simulink model "e8_IPMSM_HWJandVent_ROM"  (R2021b)
settings: Solver=VariableStepAuto  StartTime=0.0  StopTime=1000  RelTol=1e-3  AbsTol=1e-3
model workspace (MAT data in the model file):
  AdjacencyMat = [0 0 0 0 0 0 0 0 0 0 0 0 ... (15129 elements, 123x123)]
  Banding_Loss_Mat = [0 0 0 0 0 0 0 0 0 0 0 0 ... (7020 elements, 39x60x3)]
  CapMat = [1e+20; 2196.70091586; 387.653102799; 193.8265514; 1962.34710525; 387.653102799; 193.8265514; 1962.34710525; 1266.59353814; 268.053957132; 416.539515956; 175.715078; 577.243160678; 310.101557898; 23.9530731873; 15.4990473565; 47.9061463746; 30.998094713; 85.98384; 1.11955442905; 1.11955442905; 1.11955442905; 1.11955442905; 1.11955442905; 1.11955442905; 0.373184809682; 0.373184809682; 450.202206395; 54.9511679003; 54.9511679003; 247.389926005; 247.389926005; 75.306462; 75.306462; 1.11955442905; 1.11955442905; 1e+20; 1e+20; 0; 0; 0; 0; 429.469897824; 0; 0; 0; 0; 429.469897824; 0; 0; 0; 0; 0; 0; 424.408023296; 268.053957132; 0; 0; 0; 0; 0; 322.102423368; 0; 0; 0; 0; 0; 322.102423368; 0; 0; 0; 0; 0; 318.306017472; 268.053957132; 2196.70091586; 1266.59353814; 268.053957132; 416.539515956; 175.715078; 577.243160678; 310.101557898; 85.98384; 0.373184809682; 0.373184809682; 450.202206395; 0; 0; 0; 0; 0; 424.408023296; 268.053957132; 0; 0; 0; 0; 318.306017472; 268.053957132; 2196.70091586; 1266.59353814; 268.053957132; 416.539515956; 175.715078; 577.243160678; 310.101557898; 85.98384; 0.373184809682; 0.373184809682; 450.202206395; 0; 0; 0; 0; 0; 424.408023296; 268.053957132; 0; 0; 0; 0; 318.306017472; 268.053957132]
  CoolantArrayIdxs = [20; 21; 22; 23; 24; 25; 26; 27; 35; 36; 37; 84; 85; 108; 109; 19; 38; 83; 107]
  DCBusVoltageVec = [200 300 400]
  Friction_Loss_Mat = [0 0 0 0 0 0 0 0 0 0 0 0 ... (7020 elements, 39x60x3)]
  InletCoolIdxs = [38; 37]
  Iron_Loss_Rotor_Back_Iron_Mat = [0.0117705351991 0.0204390240307 0.0248508325185 0.0256457032681 0.0238785055856 0.020530699908 0.0166089076031 0.0132296142351 0.0115805086727 0.0121981902442 0.0144548234671 0.0172622621719 ... (7020 elements, 39x60x3)]
  Iron_Loss_Rotor_Pole_Mat = [1.45649756865 1.45220158629 1.42754923451 1.38825604934 1.33915333349 1.28386605183 1.22530180492 1.16593914393 1.10785564554 1.05188090135 0.997097257278 0.941639677474 ... (7020 elements, 39x60x3)]
  Iron_Loss_Rotor_Tooth_Mat = [0 0 0 0 0 0 0 0 0 0 0 0 ... (7020 elements, 39x60x3)]
  Iron_Loss_Stator_Back_Iron_Mat = [38.5419456951 37.7152025365 36.7151009719 35.6149517682 34.4520386289 33.2585547415 32.0665067995 30.91142079 29.8301048499 28.8255844376 27.8319778373 26.7434652419 ... (7020 elements, 39x60x3)]
  Iron_Loss_Stator_Tooth_Mat = [42.0610884508 40.9832240847 40.1258499541 39.3817529075 38.6582544091 37.9130136221 37.1370624807 36.3449214788 35.5617649366 34.7840580455 33.951564889 32.9872940506 ... (7020 elements, 39x60x3)]
  LossDistrForEachType = [0 0 0 0 0 0 0 0 0 0 0 0 ... (2952 elements, 24x123)]
  Magnet_Loss_Mat = [0.0995193918038 0.0923780277949 0.0864844160887 0.0815810725061 0.0772064600726 0.0729767275694 0.0685055432332 0.0633314716331 0.0569179480863 0.0491401889658 0.0406359949749 0.0323130751847 ... (7020 elements, 39x60x3)]
  OutletCoolIdxs = [107  107  107; 20  22  23]
  RotorCopperTempCoefResistivity = 0.00393
  Rotor_Cage_Loss_Mat = [0 0 0 0 0 0 0 0 0 0 0 0 ... (7020 elements, 39x60x3)]
  ShaftTorqueVec = [-286.936099977 -271.951133863 -256.966167748 -241.981201634 -226.99623552 -212.011269406 -197.026303292 -182.041337178 -167.056371063 -152.071404949 -137.086438835 -122.101472721 -107.116506607 -92.1315404924 -77.1465743783 -62.1616082641 -47.1766421499 -32.1916760357 -17.2067099215 -2.22174380736 12.7632223068 27.748188421 42.7331545352 57.7181206494 72.7030867635 87.6880528777 102.673018992 117.657985106 132.64295122 147.627917334 162.612883449 177.597849563 192.582815677 207.567781791 222.552747905 237.53771402 252.522680134 267.507646248 282.492612362]
  Sleeve_Loss_Mat = [0 0 0 0 0 0 0 0 0 0 0 0 ... (7020 elements, 39x60x3)]
  SpeedVec = [500 661.016949153 822.033898305 983.050847458 1144.06779661 1305.08474576 1466.10169492 1627.11864407 1788.13559322 1949.15254237 2110.16949153 2271.18644068 2432.20338983 2593.22033898 2754.23728814 2915.25423729 3076.27118644 3237.28813559 3398.30508475 3559.3220339 3720.33898305 3881.3559322 4042.37288136 4203.38983051 4364.40677966 4525.42372881 4686.44067797 4847.45762712 5008.47457627 5169.49152542 5330.50847458 5491.52542373 5652.54237288 5813.55932203 5974.57627119 6135.59322034 6296.61016949 6457.62711864 6618.6440678 6779.66101695 6940.6779661 7101.69491525 7262.71186441 7423.72881356 7584.74576271 7745.76271186 7906.77966102 8067.79661017 8228.81355932 8389.83050847 8550.84745763 8711.86440678 8872.88135593 9033.89830508 9194.91525424 9355.93220339 9516.94915254 9677.96610169 9838.98305085 10000]
  StateSpaceND : object (value not decoded)
  StatorCopperTempCoefResistivity = 0.00393
  Stator_Copper_Loss_AC_Mat = [0 0 0 0 0 0 0 0 0 0 0 0 ... (7020 elements, 39x60x3)]
  Stator_Copper_Loss_Mat = [3925.33912093 3478.13441392 3061.95534758 2688.26015542 2350.64396183 2044.39353286 1765.95289325 1512.57803512 1282.11615226 1072.87404999 883.521113045 712.988793321 ... (7020 elements, 39x60x3)]
  Stray_Load_Loss_Mat = [0 0 0 0 0 0 0 0 0 0 0 0 ... (7020 elements, 39x60x3)]
  Stray_Loss_Stator_Iron_Proportion = 0.95
  TnodesInit = [25; 25; 25; 25; 25; 25; 25; 25; 25; 25; 25; 25; 25; 25; 25; 25; 25; 25; 25; 25; 25; 25; 25; 25; 25; 25; 25; 25; 25; 25; 25; 25; 25; 25; 25; 25; 25; 25; 25; 25; 25; 25; 25; 25; 25; 25; 25; 25; 25; 25; 25; 25; 25; 25; 25; 25; 25; 25; 25; 25; 25; 25; 25; 25; 25; 25; 25; 25; 25; 25; 25; 25; 25; 25; 25; 25; 25; 25; 25; 25; 25; 25; 25; 25; 25; 25; 25; 25; 25; 25; 25; 25; 25; 25; 25; 25; 25; 25; 25; 25; 25; 25; 25; 25; 25; 25; 25; 25; 25; 25; 25; 25; 25; 25; 25; 25; 25; 25; 25; 25; 25; 25; 25]
  TrefRotor = 20
  TrefStator = 20
  Windage_Loss_Mat = [0 0 0 0 0 0 0 0 0 0 0 0 ... (7020 elements, 39x60x3)]
libraries: mcadROM_lib x4
(part 1 of 2)
settings Model: Creator=agonzale  LastModifiedBy=agonzale
settings SolverCC: AutoScaleAbsTol=off

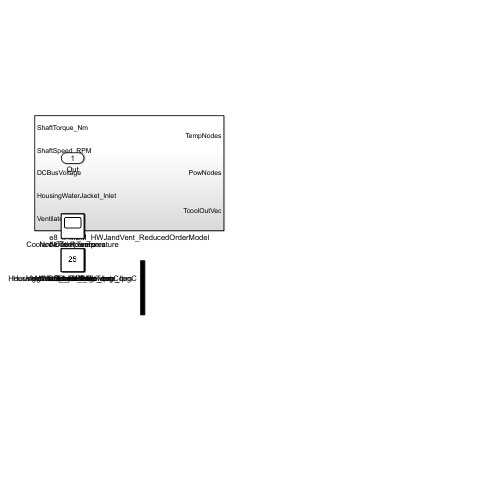
[thumbnail: Simulink's stored preview of the top-level diagram]
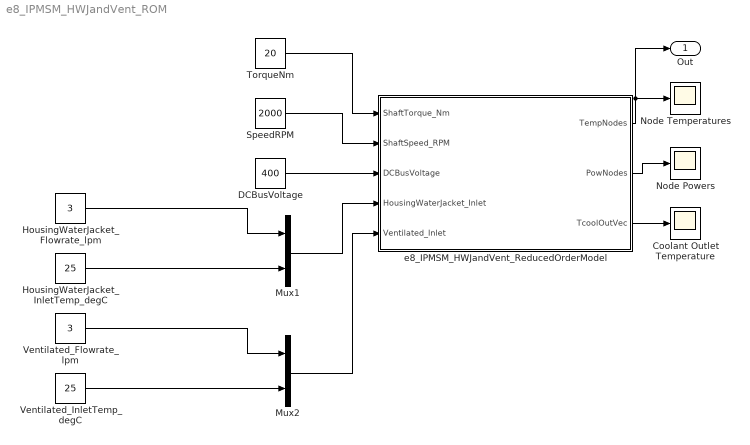
== system e8_IPMSM_HWJandVent_ROM ==
  Coolant Outlet Temperature : Scope
  DCBusVoltage : Constant  Value=400
  HousingWaterJacket_Flowrate_lpm : Constant  Value=3
  HousingWaterJacket_InletTemp_degC : Constant  Value=25
  Mux1 : Mux  Inputs=2
  Mux2 : Mux  Inputs=2
  Node Powers : Scope
  Node Temperatures : Scope
  SpeedRPM : Constant  Value=2000
  TorqueNm : Constant  Value=20
  Ventilated_Flowrate_lpm : Constant  Value=3
  Ventilated_InletTemp_degC : Constant  Value=25
  e8_IPMSM_HWJandVent_ReducedOrderModel : Subsystem
  Out : Outport
  wires:
  Ventilated_Flowrate_lpm/1 -> Mux2/1
  e8_IPMSM_HWJandVent_ReducedOrderModel/3(TcoolOutVec) -> Coolant Outlet Temperature/1
  e8_IPMSM_HWJandVent_ReducedOrderModel/2(PowNodes) -> Node Powers/1
  Mux2/1 -> e8_IPMSM_HWJandVent_ReducedOrderModel/5(Ventilated_Inlet)
  Ventilated_InletTemp_degC/1 -> Mux2/2
  Mux1/1 -> e8_IPMSM_HWJandVent_ReducedOrderModel/4(HousingWaterJacket_Inlet)
  HousingWaterJacket_InletTemp_degC/1 -> Mux1/2
  HousingWaterJacket_Flowrate_lpm/1 -> Mux1/1
  SpeedRPM/1 -> e8_IPMSM_HWJandVent_ReducedOrderModel/2(ShaftSpeed_RPM)
  DCBusVoltage/1 -> e8_IPMSM_HWJandVent_ReducedOrderModel/3(DCBusVoltage)
  TorqueNm/1 -> e8_IPMSM_HWJandVent_ReducedOrderModel/1(ShaftTorque_Nm)
  e8_IPMSM_HWJandVent_ReducedOrderModel/1(TempNodes) -> Node Temperatures/1, Out/1
